simulink model "elements"  (R2019b)
settings: Solver=VariableStepAuto  StartTime=0.0  StopTime=10.0  RelTol=1e-3
values from neighbouring files (symbols this model uses):
  a = input("Semimajor axis [km]: ")    [SCARSSetup.m]    (also in pwsat2_setup.m = 6960989.91401; pwsat2_tle.m = 6960989.91401; scars_setup.m = 6778000; startup.m = 7000000)
  e = input("Eccentricity [-]: ")    [SCARSSetup.m]    (also in pwsat2_setup.m = 0.0011871; pwsat2_tle.m = 0.0011871; scars_setup.m = 0; startup.m = 0.01)
  incl = input("Inclination [deg]: ")    [SCARSSetup.m]    (also in pwsat2_setup.m = deg2rad(97.7672); pwsat2_tle.m = deg2rad(97.7672); scars_setup.m = deg2rad(45); startup.m = deg2rad(45))
  mu = 398600.4418    [eci2kep.m]    (also in pwsat2_setup.m = 398600441800000; pwsat2_tle.m = 398600441800000; scars_setup.m = 398600441800000; startup.m = 398600441800000)
  RA = input("Right ascension of the ascending node [deg]: ")    [SCARSSetup.m]    (also in pwsat2_setup.m = deg2rad(56.1804); pwsat2_tle.m = deg2rad(56.1804); scars_setup.m = deg2rad(0); startup.m = deg2rad(10))
  TA = deg2rad(0)    [scars_setup.m]    (also in startup.m = deg2rad(10); startup_cubesat_ref.m = deg2rad(302.9234))
  w = input("Argument of periapsis [deg]: ")    [SCARSSetup.m]    (also in pwsat2_setup.m = deg2rad(236.0402); pwsat2_tle.m = deg2rad(236.0402); scars_setup.m = deg2rad(30); startup.m = deg2rad(10))
libraries: sharedutil x3
settings Model: Creator=asmialek  LastModifiedBy=asmialek

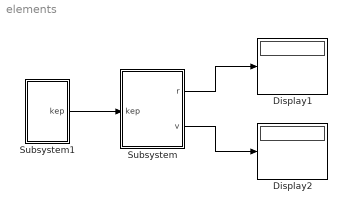
== system elements ==
  Display1 : Display
  Display2 : Display
  Subsystem : Subsystem
  Subsystem1 : Subsystem
  wires:
  Subsystem1/1(kep) -> Subsystem/1(kep)
  Subsystem/1(r) -> Display1/1
  Subsystem/2(v) -> Display2/1

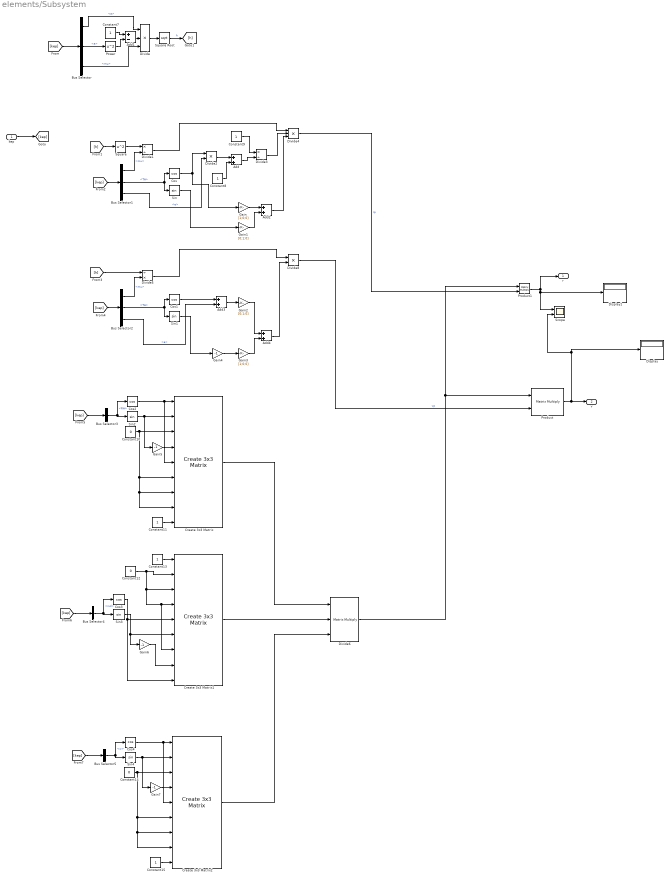
== system elements/Subsystem ==
  kep : Inport
  Add{,2..4} (4 alike) : Sum
  Add1 : Sum  Inputs=+-
  Bus Selector : BusSelector  OutputSignals=a,e,mu
  Bus Selector1 : BusSelector  OutputSignals=mu,TA,e
  Bus Selector2 : BusSelector  OutputSignals=mu,TA,e
  Bus Selector3 : BusSelector  OutputSignals=RA
  Bus Selector4 : BusSelector  OutputSignals=incl
  Bus Selector5 : BusSelector  OutputSignals=w
  Constant10 : Constant  Value=0
  Constant{7..9,11,13,15} (6 alike) : Constant
  Constant12 : Constant  Value=0
  Constant14 : Constant  Value=0
  Cos{,1..4} (5 alike) : Trigonometry  Operator=cos
  Create 3x3 Matrix : sharedutil/Create 3x3 Matrix  aMode=aMode
  Create 3x3 Matrix1 : sharedutil/Create 3x3 Matrix  aMode=aMode
  Create 3x3 Matrix2 : sharedutil/Create 3x3 Matrix  aMode=aMode
  Display : Display
  Display1 : Display
  Divide : Product  Inputs=3
  Divide1 : Product  Inputs=*/
  Divide2 : Product
  Divide3 : Product  Inputs=*/
  Divide4 : Product  Inputs=3
  Divide5 : Product  Inputs=/*
  Divide6 : Product  Inputs=3  Multiplication=Matrix(*)
  Divide8 : Product
  Gain : Gain  Gain=[1;0;0]
  Gain1 : Gain  Gain=[0;1;0]
  Gain2 : Gain  Gain=[0;1;0]
  Gain3 : Gain  Gain=[1;0;0]
  Gain{4..7} (4 alike) : Gain  Gain=-1
  Power : Math  Operator=square  SignedPower=off  SaturateOnIntegerOverflow=on
  Product : Product  Multiplication=Matrix(*)
  Product1 : Product  Multiplication=Matrix(*)
  Scope : Scope  NumInputPorts=2
  Sin{,1..4} (5 alike) : Trigonometry
  Square : Math  Operator=square  SignedPower=off  SaturateOnIntegerOverflow=on
  Square Root : Sqrt  SaturateOnIntegerOverflow=on
  r : Outport
  v : Outport  Port=2
  wires:
  Bus Selector2/1 -> Divide5/2  "<mu>"
  [h] -> Square/1
  Square Root/1 -> [h]  "h"
  Bus Selector2/3 -> Add3/2  "<e>"
  [kep] -> Bus Selector3/1
  Gain5/1 -> Create 3x3 Matrix/4
  Divide3/1 -> Divide4/2
  Constant15/1 -> Create 3x3 Matrix2/9
  Bus Selector1/1 -> Divide1/2  "<mu>"
  Gain6/1 -> Create 3x3 Matrix1/8
  Add/1 -> Divide3/2
  Create 3x3 Matrix2/1 -> Divide6/3
  Divide1/1 -> Divide4/1
  Sin1/1 -> Gain4/1
  Cos1/1 -> Add3/1
  Gain7/1 -> Create 3x3 Matrix2/4
  Gain3/1 -> Add4/2
  Cos2/1 -> Create 3x3 Matrix/5, Create 3x3 Matrix/1
  [kep] -> Bus Selector4/1
  Gain1/1 -> Add2/2
  Constant7/1 -> Add1/1
  Create 3x3 Matrix1/1 -> Divide6/2
  Divide5/1 -> Divide8/1
  Bus Selector4/1 -> Cos3/1, Sin3/1  "<incl>"
  Constant10/1 -> Create 3x3 Matrix/8, Create 3x3 Matrix/7, Create 3x3 Matrix/6, Create 3x3 Matrix/3
  Divide6/1 -> Product1/1, Product/1
  Cos3/1 -> Create 3x3 Matrix1/9, Create 3x3 Matrix1/5
  Power/1 -> Add1/2
  [kep] -> Bus Selector/1
  Constant12/1 -> Create 3x3 Matrix1/7, Create 3x3 Matrix1/4, Create 3x3 Matrix1/3, Create 3x3 Matrix1/2
  Bus Selector1/2 -> Cos/1, Sin/1  "<TA>"
  Bus Selector/3 -> Divide/3  "<mu>"
  Divide4/1 -> Product1/2  "rp"
  Bus Selector5/1 -> Cos4/1, Sin4/1  "<w>"
  Gain2/1 -> Add4/1
  Sin4/1 -> Gain7/1, Create 3x3 Matrix2/2
  Bus Selector1/3 -> Divide2/2  "<e>"
  [kep] -> Bus Selector5/1
  Gain4/1 -> Gain3/1
  Divide2/1 -> Add/1
  kep/1 -> [kep]
  [kep] -> Bus Selector1/1
  Sin3/1 -> Create 3x3 Matrix1/6, Gain6/1
  Divide8/1 -> Product/2  "vp"
  Constant13/1 -> Create 3x3 Matrix1/1
  [kep] -> Bus Selector2/1
  Bus Selector3/1 -> Cos2/1, Sin2/1  "<RA>"
  Constant8/1 -> Add/2
  Add4/1 -> Divide8/2
  Bus Selector/1 -> Divide/1  "<a>"
  Sin/1 -> Gain1/1
  Product1/1 -> r/1, Display1/1, Scope/1
  Bus Selector2/2 -> Cos1/1, Sin1/1  "<TA>"
  Add2/1 -> Divide4/3
  Add3/1 -> Gain2/1
  Constant11/1 -> Create 3x3 Matrix/9
  Constant14/1 -> Create 3x3 Matrix2/8, Create 3x3 Matrix2/7, Create 3x3 Matrix2/6, Create 3x3 Matrix2/3
  Create 3x3 Matrix/1 -> Divide6/1
  Product/1 -> v/1, Display/1, Scope/2
  Add1/1 -> Divide/2
  [h] -> Divide5/1
  Divide/1 -> Square Root/1
  Bus Selector/2 -> Power/1  "<e>"
  Cos4/1 -> Create 3x3 Matrix2/5, Create 3x3 Matrix2/1
  Sin2/1 -> Gain5/1, Create 3x3 Matrix/2
  Square/1 -> Divide1/1
  Cos/1 -> Divide2/1, Gain/1
  Constant9/1 -> Divide3/1
  Gain/1 -> Add2/1

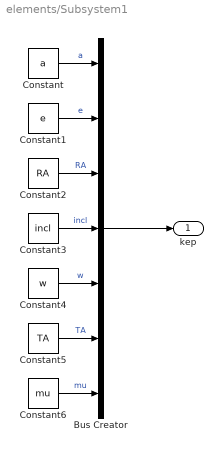
== system elements/Subsystem1 ==
  Bus Creator : BusCreator  Inputs=7
  Constant : Constant  Value=a
  Constant1 : Constant  Value=e
  Constant2 : Constant  Value=RA
  Constant3 : Constant  Value=incl
  Constant4 : Constant  Value=w
  Constant5 : Constant  Value=TA
  Constant6 : Constant  Value=mu
  kep : Outport
  wires:
  Constant4/1 -> Bus Creator/5  "w"
  Constant/1 -> Bus Creator/1  "a"
  Bus Creator/1 -> kep/1
  Constant2/1 -> Bus Creator/3  "RA"
  Constant1/1 -> Bus Creator/2  "e"
  Constant3/1 -> Bus Creator/4  "incl"
  Constant5/1 -> Bus Creator/6  "TA"
  Constant6/1 -> Bus Creator/7  "mu"
